simulink model "driveline_ctrl_est_sim"  (R2018b)
settings: Solver=ode45  StartTime=0.0  StopTime=10  MaxStep=0.001  RelTol=1e-3
values from neighbouring files (symbols this model uses):
  A = [[-ds/Jf/r^2 ds/Jf/r -cs/Jf/r];[ds/Jc/r -ds/Jc cs/Jc];[1/r -1 0]]    [drivetrain_ctrl_est_design.m]
  B1 = [B H]    [drivetrain_ctrl_est_design.m]
  B2 = [B L]    [drivetrain_ctrl_est_design.m]
  C1 = eye(3)    [drivetrain_ctrl_est_design.m]
  D = zeros(3,2)    [drivetrain_ctrl_est_design.m]
  K = P*Wrh*inv(Wr)    [drivetrain_ctrl_est_design.m]
  kr = -1/(C*inv(A-B*K)*B)    [drivetrain_ctrl_est_design.m]
  x0 = [120 2 0]'    [drivetrain_ctrl_est_design.m]
settings Model: Creator=jofr  LastModifiedBy=Csabi
settings DataIOCC: LimitDataPoints=on  SaveFormat=Array
settings OptimizationCC: BlockReduction=off  BooleanDataType=off  LifeSpan=inf
settings DebuggingCC: SaveWithParameterizedLinksMsg=none  UnderspecifiedInitializationDetection=Classic  MergeDetectMultiDrivingBlocksExec=none  SignalResolutionControl=TryResolveAllWithWarning  MultiTaskDSMMsg=warning  MultiTaskCondExecSysMsg=none  SFUnexpectedBacktrackingDiag=warning  SFNoUnconditionalDefaultTransitionDiag=warning  SFExecutionAtInitializationDiag=none
settings HardwareCC: ProdBitPerPointer=32  ProdBitPerSizeT=32  ProdBitPerPtrDiffT=32  ProdLargestAtomicFloat=None  ProdIntDivRoundTo=Undefined  ProdEndianess=Unspecified  ProdWordSize=32  ProdHWDeviceType=32-bit Generic  TargetUnknown=on
settings ModelReferenceCC: PropagateSignalLabelsOutOfModel=off
settings SFSimCC: SimUseLocalCustomCode=off
settings RTWCC: RTWUseLocalCustomCode=off
settings CodeAppCC: StateflowObjectComments=on
settings GRTTargetCC: TargetLangStandard=C89/C90 (ANSI)  GeneratePreprocessorConditionals=Disable all
settings ConfigComp: CovMetricSettings=dw  CovHtmlReporting=on  CovSaveCumulativeToWorkspaceVar=on  CovSaveSingleToWorkspaceVar=on  CovExternalEMLEnable=off

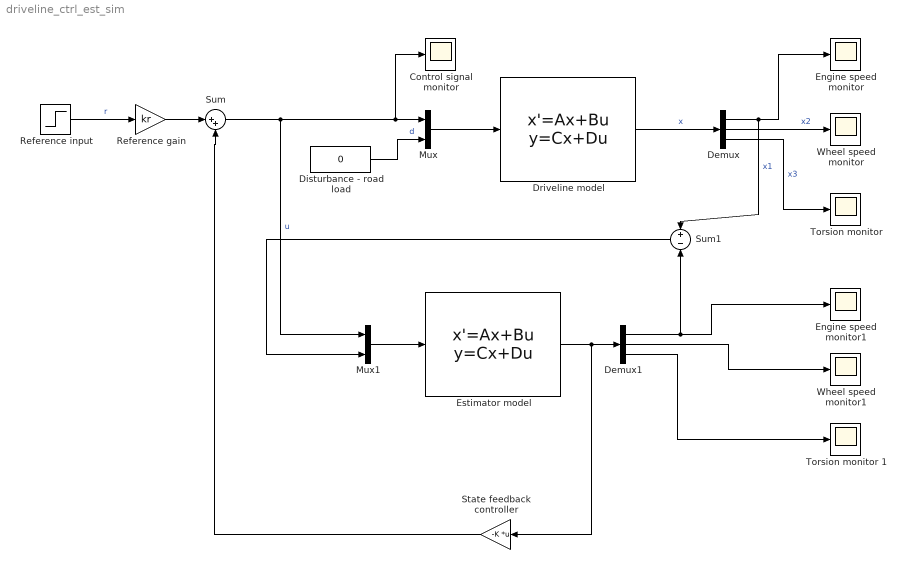
== system driveline_ctrl_est_sim ==
  Control signal monitor : Scope
  Demux : Demux  Outputs=3
  Demux1 : Demux  Outputs=3
  Disturbance - road load : Constant  Value=0
  Driveline model : StateSpace  A=A  B=B1  C=C1  D=D  InitialCondition=x0
  Engine speed monitor : Scope
  Engine speed monitor1 : Scope
  Estimator model : StateSpace  A=A  B=B2  C=C1  D=D  InitialCondition=0
  Mux : Mux  Inputs=2
  Mux1 : Mux  Inputs=2
  Reference gain : Gain  Gain=kr
  Reference input : Step  Time=4  Before=2  After=4  SampleTime=0
  State feedback controller : Gain  Gain=-K  Multiplication=Matrix(K*u)
  Sum : Sum  Inputs=|++
  Sum1 : Sum  Inputs=+|-
  "Torsion monitor " : Scope
  Torsion monitor 1 : Scope
  Wheel speed monitor : Scope
  Wheel speed monitor1 : Scope
  wires:
  Driveline model/1 -> Demux/1  "x"
  Demux/1 -> Sum1/1, Engine speed monitor/1  "x1"
  Demux/2 -> Wheel speed monitor/1  "x2"
  Demux/3 -> "Torsion monitor "/1  "x3"
  Mux/1 -> Driveline model/1
  Disturbance - road load/1 -> Mux/2  "d"
  State feedback controller/1 -> Sum/2
  Reference input/1 -> Reference gain/1  "r"
  Sum/1 -> Mux1/1, Control signal monitor/1, Mux/1  "u"
  Reference gain/1 -> Sum/1
  Mux1/1 -> Estimator model/1
  Estimator model/1 -> State feedback controller/1, Demux1/1
  Demux1/1 -> Sum1/2, Engine speed monitor1/1
  Demux1/2 -> Wheel speed monitor1/1
  Demux1/3 -> Torsion monitor 1/1
  Sum1/1 -> Mux1/2
